simulink library "Filter"  (R2018b)
settings: Solver=VariableStepAuto  StartTime=0.0  StopTime=10.0  RelTol=1e-3
undefined symbols (not defined in the file): CONTROL_CONST, DiscIntNeverNeededParam
libraries: $bdroot x1
settings Model: Creator=zouji  LastModifiedBy=zouji

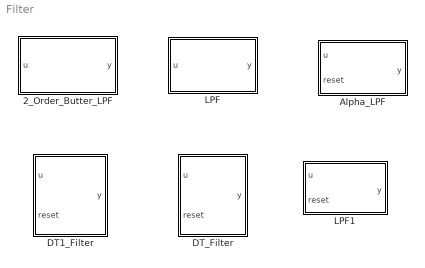
== system Filter ==
  2_Order_Butter_LPF : Subsystem  mask{wn=30*2*pi, ksi=0.707}
      mask prompts: wn "Cut Frequency (rad/s)"; ksi "Damping Ratio"
  Alpha_LPF : Subsystem  mask{wn=0, dt=0}
      mask prompts: wn "Cut-off freq (Hz)"; dt "dT (s)"
  DT1_Filter : Subsystem  mask{wn=0}
      mask prompts: wn "Cut-off freq [Hz]"
      mask Display: fprintf('Wn = %.1f', wn)
  DT_Filter : Subsystem  mask{wn=0}
      mask prompts: wn "Cut-off freq (Hz)"
      mask Display: fprintf('wn = %d Hz', wn)
  LPF : Subsystem  mask{T=0}
      mask prompts: T "Time Constant (s)"
  LPF1 : Subsystem  mask{wn=0, dt=0}
      mask prompts: wn "Cutoff Frequency (Hz)"

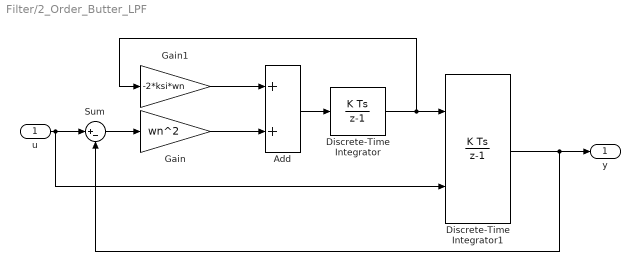
== system Filter/2_Order_Butter_LPF ==
  u : Inport
  Add : Sum
  Discrete-Time Integrator : DiscreteIntegrator  SampleTime=-1  ICPrevOutput=DiscIntNeverNeededParam  ICPrevScaledInput=DiscIntNeverNeededParam
  Discrete-Time Integrator1 : DiscreteIntegrator  InitialConditionSource=external  SampleTime=-1  ICPrevOutput=DiscIntNeverNeededParam  ICPrevScaledInput=DiscIntNeverNeededParam
  Gain : Gain  Gain=wn^2
  Gain1 : Gain  Gain=-2*ksi*wn
  Sum : Sum  Inputs=|+-
  y : Outport
  wires:
  Gain1/1 -> Add/1
  Add/1 -> Discrete-Time Integrator/1
  Sum/1 -> Gain/1
  Gain/1 -> Add/2
  Discrete-Time Integrator1/1 -> Sum/2, y/1
  Discrete-Time Integrator/1 -> Gain1/1, Discrete-Time Integrator1/1
  u/1 -> Discrete-Time Integrator1/2, Sum/1

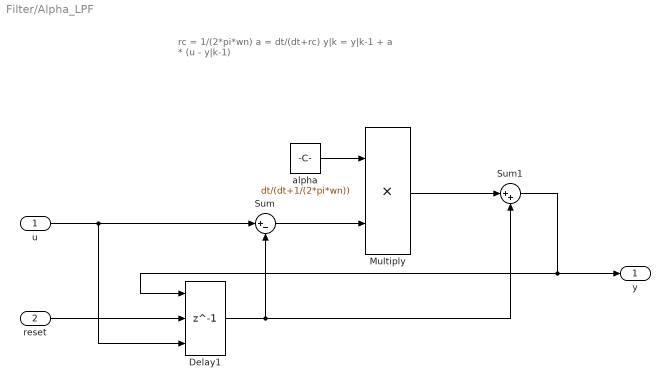
== system Filter/Alpha_LPF ==
  note: rc = 1/(2*pi*wn)
      | a = dt/(dt+rc)
      |
      | y|k = y|k-1 + a * (u - y|k-1)
  u : Inport
  reset : Inport  Port=2
  Delay1 : Delay  DelayLength=1  InitialConditionSource=Input port  ExternalReset=Level
      settings: InputPortMap=u0,r5,p4
  Multiply : Product
  Sum : Sum  Inputs=|+-
  Sum1 : Sum  Inputs=|++
  alpha : Constant  Value=dt/(dt+1/(2*pi*wn))  OutDataTypeStr=single
  y : Outport
  wires:
  Delay1/1 -> Sum/2, Sum1/2
  u/1 -> Delay1/3, Sum/1
  reset/1 -> Delay1/2
  alpha/1 -> Multiply/1
  Sum/1 -> Multiply/2
  Multiply/1 -> Sum1/1
  Sum1/1 -> Delay1/1, y/1

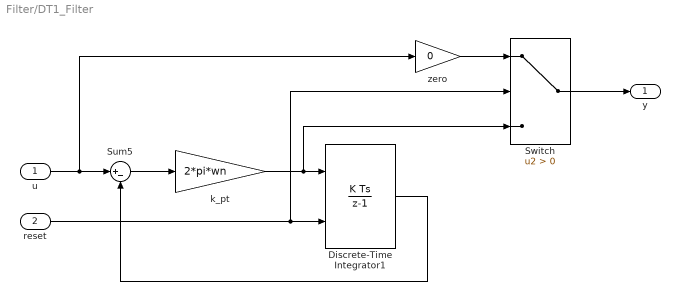
== system Filter/DT1_Filter ==
  u : Inport
  reset : Inport  Port=2
  Discrete-Time Integrator1 : DiscreteIntegrator  ExternalReset=level  SampleTime=-1  ICPrevOutput=DiscIntNeverNeededParam  ICPrevScaledInput=DiscIntNeverNeededParam
  Sum5 : Sum  Inputs=|+-
  Switch : Switch  Criteria=u2 > Threshold
  k_pt : Gain  Gain=2*pi*wn  OutDataTypeStr=Inherit: Same as input
  zero : Gain  Gain=0  OutDataTypeStr=Inherit: Same as input
  y : Outport
  wires:
  Sum5/1 -> k_pt/1
  Discrete-Time Integrator1/1 -> Sum5/2
  k_pt/1 -> Switch/3, Discrete-Time Integrator1/1
  Switch/1 -> y/1
  u/1 -> zero/1, Sum5/1
  reset/1 -> Switch/2, Discrete-Time Integrator1/2
  zero/1 -> Switch/1

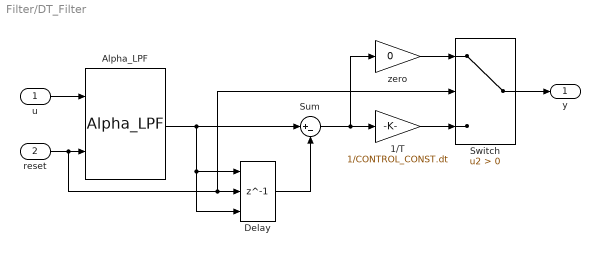
== system Filter/DT_Filter ==
  u : Inport
  reset : Inport  Port=2
  1/T : Gain  Gain=1/CONTROL_CONST.dt  OutDataTypeStr=Inherit: Same as input
  Alpha_LPF : $bdroot/Alpha_LPF  wn=wn  dt=CONTROL_CONST.dt
  Delay : Delay  DelayLength=1  InitialConditionSource=Input port  ExternalReset=Level
      settings: InputPortMap=u0,r5,p4
  Sum : Sum  Inputs=|+-
  Switch : Switch  Criteria=u2 > Threshold
  zero : Gain  Gain=0  OutDataTypeStr=Inherit: Same as input
  y : Outport
  wires:
  1/T/1 -> Switch/3
  Sum/1 -> zero/1, 1/T/1
  Alpha_LPF/1 -> Sum/1, Delay/1, Delay/3
  Delay/1 -> Sum/2
  u/1 -> Alpha_LPF/1
  reset/1 -> Switch/2, Delay/2, Alpha_LPF/2
  Switch/1 -> y/1
  zero/1 -> Switch/1

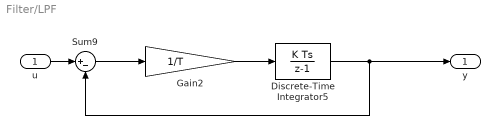
== system Filter/LPF ==
  u : Inport
  Discrete-Time Integrator5 : DiscreteIntegrator  SampleTime=-1  OutDataTypeStr=single  UpperSaturationLimit=20/180*pi  LowerSaturationLimit=-20/180*pi  ICPrevOutput=DiscIntNeverNeededParam  ICPrevScaledInput=DiscIntNeverNeededParam
  Gain2 : Gain  Gain=1/T
  Sum9 : Sum  Inputs=|+-
  y : Outport
  wires:
  u/1 -> Sum9/1
  Sum9/1 -> Gain2/1
  Discrete-Time Integrator5/1 -> y/1, Sum9/2
  Gain2/1 -> Discrete-Time Integrator5/1

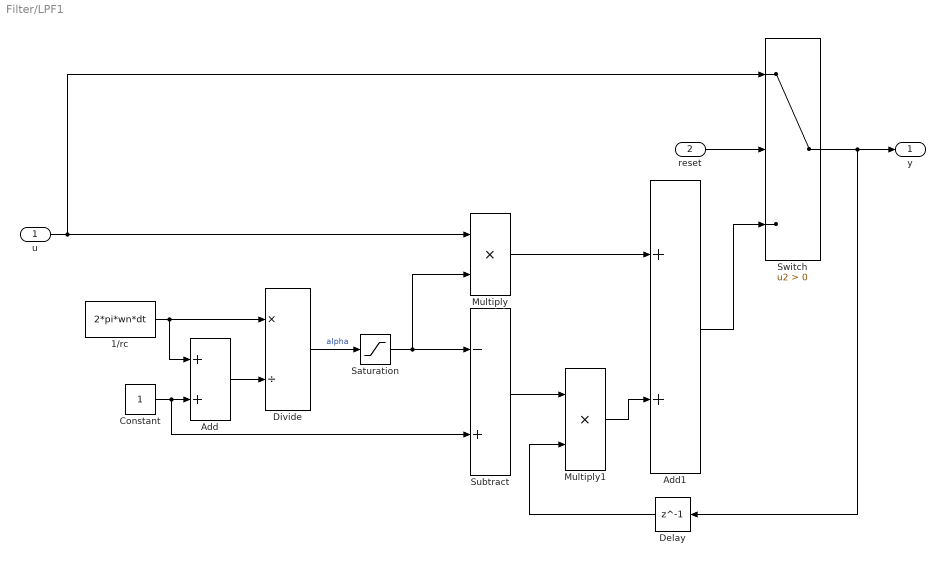
== system Filter/LPF1 ==
  u : Inport
  reset : Inport  Port=2
  1/rc : Constant  Value=2*pi*wn*dt  OutDataTypeStr=single
  Add : Sum
  Add1 : Sum
  Constant : Constant  OutDataTypeStr=single
  Delay : Delay  DelayLength=1
  Divide : Product  Inputs=*/
  Multiply : Product
  Multiply1 : Product
  Saturation : Saturate  UpperLimit=1  LowerLimit=0
  Subtract : Sum  Inputs=-+
  Switch : Switch  Criteria=u2 > Threshold
  y : Outport
  wires:
  1/rc/1 -> Add/1, Divide/1
  Add/1 -> Divide/2
  Constant/1 -> Subtract/2, Add/2
  Divide/1 -> Saturation/1  "alpha"
  u/1 -> Multiply/1, Switch/1
  Saturation/1 -> Subtract/1, Multiply/2
  Delay/1 -> Multiply1/2
  Subtract/1 -> Multiply1/1
  Multiply/1 -> Add1/1
  Multiply1/1 -> Add1/2
  reset/1 -> Switch/2
  Add1/1 -> Switch/3
  Switch/1 -> Delay/1, y/1
